simulink model "BlockDiagramNotReduced"  (R2024a)
settings: Solver=VariableStepAuto  StartTime=0.0  StopTime=10.0  RelTol=1e-3
values from neighbouring files (symbols this model uses):
  a1 = mw*Lw^2+If    (= 0.00856208)    [SystemVariablesForTransferFunction.m]
  a2 = (mf*Lf+mw*Lw)*g    (= 0.712409576)    [SystemVariablesForTransferFunction.m]
  Bf = 0.0036    [SystemVariablesForTransferFunction.m]
  Bw = 1.93*10^(-5)    (= 1.93e-05)    [SystemVariablesForTransferFunction.m]
  Iw = 699*10^(-6)    (= 0.000699)    [SystemVariablesForTransferFunction.m]
settings Model: Creator=dexti  LastModifiedBy=gusta
settings RTWCC: GPUComputeCapability=3.5

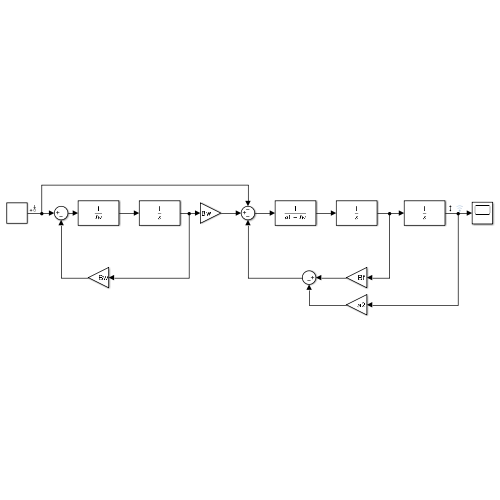
[thumbnail: Simulink's stored preview of the top-level diagram]
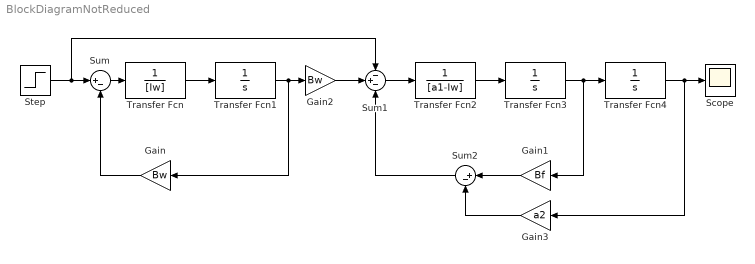
== system BlockDiagramNotReduced ==
  Gain : Gain  Gain=Bw
  Gain1 : Gain  Gain=Bf
  Gain2 : Gain  Gain=Bw
  Gain3 : Gain  Gain=a2
  Scope : Scope
  Step : Step  SampleTime=0
  Sum : Sum  Inputs=|+-
  Sum1 : Sum  Inputs=-+-
  Sum2 : Sum  Inputs=|+-
  Transfer Fcn : TransferFcn  Denominator=[Iw]
  Transfer Fcn1 : TransferFcn  Denominator=[1 0]
  Transfer Fcn2 : TransferFcn  Denominator=[a1-Iw]
  Transfer Fcn3 : TransferFcn  Denominator=[1 0]
  Transfer Fcn4 : TransferFcn  Denominator=[1 0]
  wires:
  Sum/1 -> Transfer Fcn/1
  Transfer Fcn/1 -> Transfer Fcn1/1
  Transfer Fcn1/1 -> Gain/1, Gain2/1
  Gain2/1 -> Sum1/2
  Transfer Fcn2/1 -> Transfer Fcn3/1
  Gain3/1 -> Sum2/2
  Gain1/1 -> Sum2/1
  Sum2/1 -> Sum1/3
  Sum1/1 -> Transfer Fcn2/1
  Step/1 -> Sum1/1, Sum/1
  Gain/1 -> Sum/2
  Transfer Fcn3/1 -> Gain1/1, Transfer Fcn4/1
  Transfer Fcn4/1 -> Gain3/1, Scope/1
